simulink model "SimuLinkD1SL"  (R2025b)
settings: Solver=ode4  StartTime=0.0  StopTime=110  FixedStep=1e-3  RelTol=1e-3
settings Model: Creator=luketucker  LastModifiedBy=luketucker

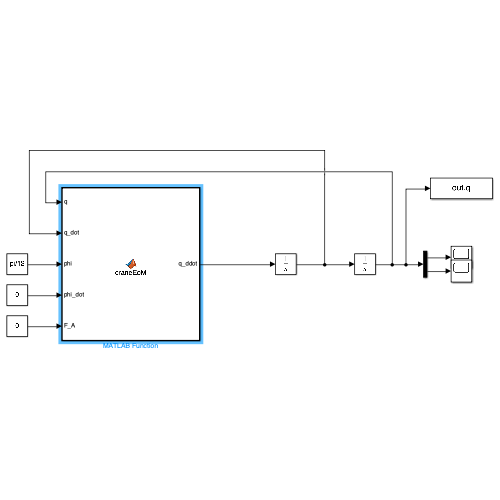
[thumbnail: Simulink's stored preview of the top-level diagram]
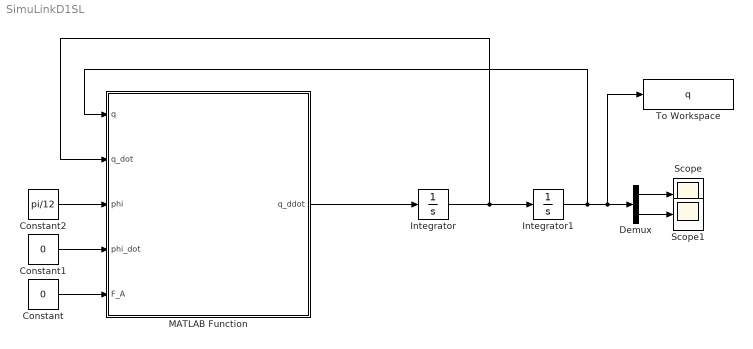
== system SimuLinkD1SL ==
  Constant : Constant  Value=0
  Constant1 : Constant  Value=0
  Constant2 : Constant  Value=pi/12
  Demux : Demux  Outputs=2
  Integrator : Integrator  InitialCondition=[0;0]
  Integrator1 : Integrator  InitialCondition=[11.5;pi/3]
  MATLAB Function : MATLAB Function  TreatAsAtomicUnit=on
  Scope : Scope
      settings: ActiveDisplayYMinimum=-1  ActiveDisplayYMaximum=1
  Scope1 : Scope
      settings: ActiveDisplayYMinimum=-1  ActiveDisplayYMaximum=1
  To Workspace : ToWorkspace  VariableName=q  SampleTime=-1
  wires:
  MATLAB Function/1(q_ddot) -> Integrator/1
  Integrator/1 -> Integrator1/1, MATLAB Function/2(q_dot)
  Integrator1/1 -> To Workspace/1, Demux/1, MATLAB Function/1(q)
  Constant/1 -> MATLAB Function/5(F_A)
  Constant1/1 -> MATLAB Function/4(phi_dot)
  Constant2/1 -> MATLAB Function/3(phi)
  Demux/1 -> Scope/1
  Demux/2 -> Scope1/1

== matlab function SimuLinkD1SL/MATLAB Function ==
  data: q input; q_ddot output; q_dot input; phi input; phi_dot input; F_A input
 function q_ddot = craneEoM(q, q_dot, phi, phi_dot, F_A)

    %Constants
    g = 9.81;

    %Masses
    m_0 = 1e4;
    m_1 = 1e4;
    m_2 = 2e3;
    m_3 = 500;

    %Lengths
    L_0 = 30;
    L_1 = 25;
    L_2 = 10; 
    L_x = 12.5; 

    %Damping 
    d_x = 200;
    d_W = 2000;
    d_phi = 2;
    k_theta = 200;
    theta_ref = 0;
    d_theta = 10;
    k_x = 7000;

    %Generalized coordinates
    x          = q(1);
    theta      = q(2);
    x_dot      = q_dot(1);
    theta_dot  = q_dot(2);

    %Mass matrix M
    %M = [m_2 + m_3,             -L_2*m_3*sin(phi - theta);
     %-L_2*m_3*sin(phi - theta),  L_2^2*m_3];

    %Forcing vector F(q, q_dot, phi, phi_dot, phi_ddot, t)

    %F1 = F_A ...
     %- d_x*x_dot ...
     %+ m_3*( 2*x*phi_dot^2 + cos(phi - theta)*phi_dot )/2 ...
     %+ k_x*( 2*L_x - 2*x )/2 ...
     %+ m_2*phi_dot^2*x ...
     %- g*m_2*sin(phi)/2 ...
     %- g*m_3*sin(phi) ...
     %- d_W*theta_dot*( sin(phi)*sin(theta) - cos(theta)^2 ) ...
     %- L_2*m_3*theta_dot^2*cos(phi - theta) ...
     %+ L_2*m_3*phi_dot*theta_dot*cos(phi - theta);

    %F2 = d_theta*(phi_dot - theta_dot) ...
     %+ k_theta*( 2*phi - 2*theta )/2 ...
     %+ L_2*g*m_3*cos(theta) ...
     %+ L_2*d_W*theta_dot*sin(2*theta) ...
     %+ m_3*phi_dot*x*sin(phi - theta)/2 ...
     %+ L_2*m_3*phi_dot*x_dot*cos(phi - theta);

    %F = [F1; F2];

    %Solve for qdd 
    %q_ddot = M \ F;     % 2x1 output: [x_ddot; theta_ddot]

    % Call auto-generated symbolic functions
    M = craneM_sym( x, theta, x_dot, theta_dot, ...
                    phi, phi_dot, F_A, ...
                    g, m_0, m_1, m_2, m_3, ...
                    L_0, L_1, L_2, L_x, ...
                    d_x, d_W, d_phi, k_theta, theta_ref, d_theta, k_x );

    F = craneF_sym( x, theta, x_dot, theta_dot, ...
                    phi, phi_dot, F_A, ...
                    g, m_0, m_1, m_2, m_3, ...
                    L_0, L_1, L_2, L_x, ...
                    d_x, d_W, d_phi, k_theta, theta_ref, d_theta, k_x );

    % Solve for accelerations
    q_ddot = M \ F;     % 2x1: [x_ddot; theta_ddot]




end
